simulink library "newton"  (R2023a)
settings: Solver=VariableStepAuto  StartTime=0.0  StopTime=10.0  RelTol=1e-3
undefined symbols (not defined in the file): b, d, D_rot, D_transl, eulerlimit, g, J1, J2, J3, Jr, L, m, R
settings Model: Creator=Alex  LastModifiedBy=Alex

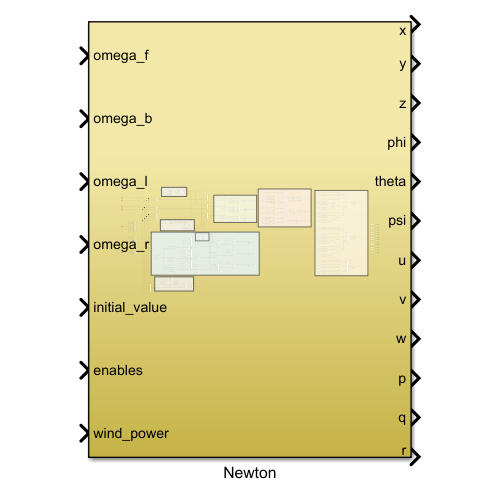
[thumbnail: Simulink's stored preview of the top-level diagram]
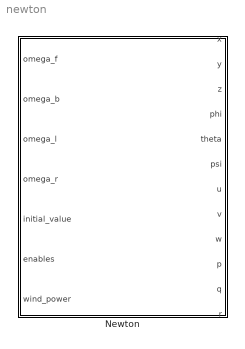
== system newton ==
  Newton : Subsystem

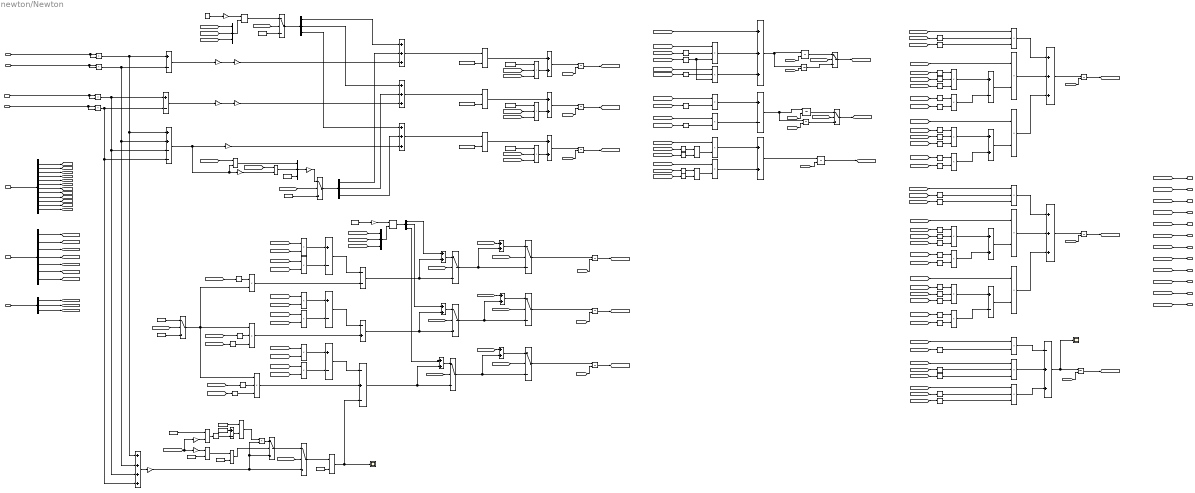
== system newton/Newton ==
  note: Drag force
  note: Ground
  note: Drag torque
  note: Gyro
  note: Inertial velocities in terms of body fixed velocities
      | Translational velocities
  note: Newton's second law
      | Translational accelerations
  note: Euler Angles
      | Rotational velocities
  note: Euler equations of motion
      | Rotational accelerations
  omega_f : Inport
  omega_b : Inport  Port=2
  omega_l : Inport  Port=3
  omega_r : Inport  Port=4
  initial_value : Inport  Port=5
  enables : Inport  Port=6
  wind_power : Inport  Port=7
  Add{,1,8,15..17,19,23,26} (9 alike) : Sum  Inputs=+-
  Add{7,10..11,18,21,25} (6 alike) : Sum  Inputs=+++
  Add12 : Sum  Inputs=--
  Add13 : Sum  Inputs=-+
  Add14 : Sum  Inputs=-+-
  Add2 : Sum  Inputs=++--
  Add{3..5,9,20,22,27..32} (12 alike) : Sum
  Add24 : Sum  Inputs=-++
  Add6 : Sum  Inputs=++++
  Constant : Constant  Value=J1
  Constant1 : Constant  Value=J2
  Constant10 : Constant  Value=R
  Constant{7,9,11,13} (4 alike) : Constant  Value=0
  Constant12 : Constant  Value=D_rot
  Constant14 : Constant  Value=0.25
  Constant15 : Constant  Value=R
  Constant16 : Constant
  Constant17 : Constant
  Constant18 : Constant  Value=D_transl
  Constant2 : Constant  Value=J3
  Constant3 : Constant  Value=(J2-J3)/J1
  Constant4 : Constant  Value=(J3-J1)/J2
  Constant5 : Constant  Value=(J1-J2)/J3
  Constant6 : Constant  Value=m
  Constant8 : Constant  Value=g
  Cos10 : Trigonometry
  Cos{2..8,11..12} (9 alike) : Trigonometry  Operator=cos
  Cos13 : Trigonometry
  Cos9 : Trigonometry
  Demux : Demux  Outputs=12
  Demux1 : Demux  Outputs=7
  Demux{2..5} (4 alike) : Demux  Outputs=3
  Divide{,1..8} (9 alike) : Product  Inputs=*/
  Gain : Gain  Gain=b
  Gain1 : Gain  Gain=L
  Gain10 : Gain  Gain=4
  Gain{6,8..9,11} (4 alike) : Gain  Gain=-1
  Gain2 : Gain  Gain=b
  Gain3 : Gain  Gain=L
  Gain4 : Gain  Gain=d
  Gain5 : Gain  Gain=b
  Gain7 : Gain  Gain=Jr
  Integrator{,1..3,6..7,9..13} (11 alike) : Integrator  InitialConditionSource=external
  Integrator4 : Integrator  InitialConditionSource=external  LimitOutput=on  UpperSaturationLimit=eulerlimit  LowerSaturationLimit=-eulerlimit
  Integrator5 : Integrator  InitialConditionSource=external  LimitOutput=on  UpperSaturationLimit=eulerlimit  LowerSaturationLimit=-eulerlimit
  Integrator8 : Integrator  InitialConditionSource=external  LimitOutput=on  UpperSaturationLimit=pi  LowerSaturationLimit=-pi
  Mux : Mux  Inputs=3
  Mux1 : Mux  Inputs=3
  Mux2 : Mux  Inputs=3
  Product{,1..3,9..13,17..19,21..26,28..29,31,33,35..36,38,40,42} (27 alike) : Product
  Product{4..8,14..15,27,30,32,34,37,39,41,43} (15 alike) : Product  Inputs=3
  Product16 : Product  Multiplication=Matrix(*)
  Product20 : Product  Multiplication=Matrix(*)
  Relational Operator : RelationalOperator  Operator=>  OutDataTypeStr=boolean  RndMeth=Simplest  InputSameDT=off
  Scope1 : Scope
  Scope6 : Scope
  Sin{,3..4,8,10,12..19,21..22,24..25} (17 alike) : Trigonometry
  Sin{1..2,5..7,9,11,20,23,26..29} (13 alike) : Trigonometry  Operator=cos
  Square : Math  Operator=square
  Switch{,1..12} (13 alike) : Switch  Criteria=u2 ~= 0  SaturateOnIntegerOverflow=off  InputSameDT=off
  Tan : Trigonometry  Operator=tan
  x : Outport
  y : Outport  Port=2
  z : Outport  Port=3
  phi : Outport  Port=4
  theta : Outport  Port=5
  psi : Outport  Port=6
  u : Outport  Port=7
  v : Outport  Port=8
  w : Outport  Port=9
  p : Outport  Port=10
  q : Outport  Port=11
  r : Outport  Port=12
  wires:
  omega_l/1 -> Product/2, Product/1
  omega_r/1 -> Product1/2, Product1/1
  Product/1 -> Add6/1, Add2/1, Add/1
  Product1/1 -> Add6/2, Add2/2, Add/2
  Add/1 -> Gain/1
  Gain/1 -> Gain1/1
  Gain1/1 -> Add25/3  "M1"
  Gain3/1 -> Add11/3  "M2"
  Gain2/1 -> Gain3/1
  Add1/1 -> Gain2/1
  Product3/1 -> Add1/2, Add6/4, Add2/4
  Product2/1 -> Add1/1, Add6/3, Add2/3
  omega_b/1 -> Product3/2, Product3/1
  omega_f/1 -> Product2/2, Product2/1
  Add2/1 -> Gain8/1, Product17/2, Gain4/1
  Gain4/1 -> Add10/3  "M3"
  Constant/1 -> Divide/2
  Constant1/1 -> Divide1/2
  Constant2/1 -> Divide2/2
  Divide/1 -> Add3/1
  Divide1/1 -> Add4/1
  Divide2/1 -> Add5/1
  Integrator/1 -> [p]  "p"
  Integrator1/1 -> [q]  "q"
  Integrator2/1 -> [r]  "r"
  Product4/1 -> Add3/2
  Product5/1 -> Add4/2
  Product6/1 -> Add5/2
  Constant3/1 -> Product4/1
  Constant4/1 -> Product5/1
  Constant5/1 -> Product6/1
  Add3/1 -> Integrator/1
  Add4/1 -> Integrator1/1
  Add5/1 -> Integrator2/1
  [q] -> Product4/2
  [r] -> Product4/3
  [r] -> Product5/2
  [p] -> Product5/3
  [p] -> Product6/2
  [q] -> Product6/3
  Add6/1 -> Gain5/1
  Gain5/1 -> Product19/2, Switch4/3, Switch2/3  "Fa"
  [p] -> Add7/1
  Product7/1 -> Add7/2
  Product8/1 -> Add7/3
  [phi] -> Sin/1
  Sin/1 -> Product7/2
  [theta] -> Tan/1
  Tan/1 -> Product8/3, Product7/3
  [phi] -> Sin1/1
  Sin1/1 -> Product8/2
  [r] -> Product8/1
  [phi] -> Sin2/1
  Sin2/1 -> Product9/2
  [q] -> Product9/1
  Product9/1 -> Add8/1
  Product10/1 -> Add8/2
  [r] -> Product10/1
  [phi] -> Sin3/1
  Sin3/1 -> Product10/2
  Divide3/1 -> Product11/2
  [q] -> Product11/1
  [r] -> Product12/1
  [phi] -> Sin4/1
  Sin4/1 -> Divide3/1
  Sin5/1 -> Divide3/2
  [theta] -> Sin5/1
  Product11/1 -> Add9/1
  Product12/1 -> Add9/2
  Divide4/1 -> Product12/2
  [phi] -> Sin6/1
  Sin6/1 -> Divide4/1
  Sin7/1 -> Divide4/2
  [theta] -> Sin7/1
  Constant6/1 -> Divide5/2
  Product14/1 -> Add13/2
  Product13/1 -> Add12/2
  Product21/1 -> Add15/1
  Product22/1 -> Add15/2
  Add15/1 -> Add12/1
  Switch10/1 -> Integrator12/1
  Integrator12/1 -> [u]  "u"
  Switch9/1 -> Integrator6/1
  Integrator6/1 -> [v]  "v"
  Integrator7/1 -> [w]  "w"
  [w] -> Product21/2
  [q] -> Product21/1
  [r] -> Product22/1
  [v] -> Product22/2
  Add16/1 -> Add13/1
  [w] -> Product24/2
  [p] -> Product24/1
  [r] -> Product23/1
  [u] -> Product23/2
  Product24/1 -> Add16/2
  Product23/1 -> Add16/1
  Product25/1 -> Add17/1
  Product26/1 -> Add17/2
  [v] -> Product25/2
  [p] -> Product25/1
  [q] -> Product26/1
  [u] -> Product26/2
  Add17/1 -> Add14/1
  Product28/1 -> Add18/2
  Product27/1 -> Add18/1
  Product29/1 -> Add18/3
  [u] -> Product27/1
  [v] -> Product28/1
  [w] -> Product29/1
  Integrator10/1 -> [x]
  Add19/1 -> Product28/2
  Add20/1 -> Product29/2
  [theta] -> Cos2/1
  Cos2/1 -> Product27/2
  [psi] -> Cos3/1
  Cos3/1 -> Product27/3
  Product30/1 -> Add19/1
  Sin12/1 -> Product30/1
  [phi] -> Sin12/1
  Sin13/1 -> Product30/2
  [theta] -> Sin13/1
  [psi] -> Cos4/1
  Cos4/1 -> Product30/3
  Product31/1 -> Add19/2
  Sin14/1 -> Product31/2
  [phi] -> Cos5/1
  [psi] -> Sin14/1
  Cos5/1 -> Product31/1
  Product32/1 -> Add20/1
  Product33/1 -> Add20/2
  Cos6/1 -> Product32/1
  Sin15/1 -> Product32/2
  Cos7/1 -> Product32/3
  [phi] -> Cos6/1
  [theta] -> Sin15/1
  [psi] -> Cos7/1
  Sin16/1 -> Product33/1
  Sin17/1 -> Product33/2
  [phi] -> Sin16/1
  [psi] -> Sin17/1
  [psi] -> Sin23/1
  [phi] -> Sin22/1
  Sin23/1 -> Product40/2
  Sin22/1 -> Product40/1
  [psi] -> Cos13/1
  [theta] -> Sin21/1
  [phi] -> Cos12/1
  Cos13/1 -> Product39/3
  Sin21/1 -> Product39/2
  Cos12/1 -> Product39/1
  Product40/1 -> Add23/2
  Product39/1 -> Add23/1
  Cos11/1 -> Product38/1
  [psi] -> Sin20/1
  [phi] -> Cos11/1
  Sin20/1 -> Product38/2
  Product38/1 -> Add22/2
  Cos10/1 -> Product37/3
  [psi] -> Cos10/1
  [theta] -> Sin19/1
  Sin19/1 -> Product37/2
  [phi] -> Sin18/1
  Sin18/1 -> Product37/1
  Product37/1 -> Add22/1
  Cos9/1 -> Product34/3
  [psi] -> Cos9/1
  Cos8/1 -> Product34/2
  [theta] -> Cos8/1
  Add23/1 -> Product36/2
  Add22/1 -> Product35/2
  Integrator11/1 -> [y]
  [w] -> Product36/1
  [v] -> Product35/1
  [u] -> Product34/1
  Product36/1 -> Add21/3
  Product34/1 -> Add21/1
  Product35/1 -> Add21/2
  Add24/1 -> Integrator3/1, Scope6/1
  Integrator3/1 -> [z]
  Product41/1 -> Add24/3
  Product43/1 -> Add24/2
  Product42/1 -> Add24/1
  [theta] -> Sin24/1
  [u] -> Product42/1
  Sin24/1 -> Product42/2
  [v] -> Product43/1
  [w] -> Product41/1
  [phi] -> Sin27/1
  [theta] -> Sin28/1
  [phi] -> Sin25/1
  [theta] -> Sin26/1
  Sin25/1 -> Product43/2
  Sin26/1 -> Product43/3
  Sin27/1 -> Product41/2
  Sin28/1 -> Product41/3
  [x] -> x/1
  [y] -> y/1
  [r] -> r/1
  [q] -> q/1
  [p] -> p/1
  [w] -> w/1
  [v] -> v/1
  [u] -> u/1
  [psi] -> psi/1
  [theta] -> theta/1
  [phi] -> phi/1
  [z] -> z/1
  Divide5/1 -> Scope1/1, Add14/3
  [q] -> Product7/1
  [theta] -> Sin8/1
  Sin8/1 -> Product13/1
  Switch/1 -> Product14/1, Product13/2, Product15/1  "gravity"
  [theta] -> Sin9/1
  Sin9/1 -> Product14/2
  [phi] -> Sin10/1
  Sin10/1 -> Product14/3
  Product15/1 -> Add14/2
  [theta] -> Sin11/1
  Sin11/1 -> Product15/2
  Sin29/1 -> Product15/3
  [phi] -> Sin29/1
  initial_value/1 -> Demux/1
  Demux/1 -> [x0]
  Demux/2 -> [y0]
  Demux/3 -> [z0]
  Demux/4 -> [phi0]
  Demux/5 -> [theta0]
  Demux/6 -> [psi0]
  Demux/7 -> [u0]
  Demux/8 -> [v0]
  Demux/9 -> [w0]
  Demux/10 -> [p0]
  Demux/11 -> [q0]
  Demux/12 -> [r0]
  [p0] -> Integrator/2
  [q0] -> Integrator1/2
  [r0] -> Integrator2/2
  [u0] -> Integrator12/2
  [v0] -> Integrator6/2
  [w0] -> Integrator7/2
  Switch8/1 -> Integrator7/1
  [z0] -> Integrator3/2
  [y0] -> Integrator11/2
  Add21/1 -> Integrator11/1
  Add18/1 -> Integrator10/1
  [x0] -> Integrator10/2
  enables/1 -> Demux1/1
  Demux1/1 -> [Ena_gravity]
  Demux1/3 -> [Ena_gyro]
  Demux1/4 -> [Ena_ground]
  Demux1/5 -> [Ena_drag_force]
  Demux1/6 -> [Ena_drag_torque]
  Demux1/7 -> [Ena_wind]
  wind_power/1 -> Demux5/1
  [Ena_gravity] -> Switch/2
  Constant8/1 -> Switch/1
  Constant7/1 -> Switch/3
  Add10/1 -> Divide2/1  "tau3"
  Add11/1 -> Divide1/1  "tau2"
  Add25/1 -> Divide/1  "tau1"
  [Ena_gyro] -> Switch1/2
  [Ena_drag_torque] -> Switch3/2
  Constant9/1 -> Switch3/3
  Constant11/1 -> Switch1/3
  Constant12/1 -> Gain6/1
  Gain6/1 -> Product16/1
  [q] -> Mux/2
  [p] -> Mux/1
  [r] -> Mux/3
  Mux/1 -> Product16/2
  Product16/1 -> Switch3/1
  Switch3/1 -> Demux2/1  "drag_torque"
  Switch1/1 -> Demux3/1  "gyro"
  [q] -> Product17/1
  [p] -> Product18/1
  Product17/1 -> Mux1/1
  Product18/1 -> Mux1/2
  Constant13/1 -> Mux1/3
  Mux1/1 -> Gain7/1
  Gain7/1 -> Switch1/1
  Gain8/1 -> Product18/2
  Demux3/3 -> Add10/2
  Demux3/2 -> Add11/2
  Demux3/1 -> Add25/2
  Demux2/2 -> Add11/1
  [Ena_ground] -> Switch2/2
  Switch2/1 -> Divide5/1  "ground"
  Switch4/1 -> Switch2/1
  [z] -> Gain10/1, Gain9/1
  Gain9/1 -> Divide6/1
  Divide6/1 -> Relational Operator/1
  Constant10/1 -> Divide6/2
  Relational Operator/1 -> Switch4/2
  Constant14/1 -> Relational Operator/2
  Product19/1 -> Switch4/1
  Constant15/1 -> Divide7/1
  Gain10/1 -> Divide7/2
  Divide7/1 -> Square/1
  Square/1 -> Add26/2
  Constant16/1 -> Add26/1
  Divide8/1 -> Product19/1
  Add26/1 -> Divide8/2
  Constant17/1 -> Divide8/1
  [Ena_drag_force] -> Switch5/2
  Add14/1 -> Add27/2, Switch5/3
  Add27/1 -> Switch5/1
  Mux2/1 -> Product20/2
  [w] -> Mux2/3
  [u] -> Mux2/1
  Gain11/1 -> Product20/1
  Constant18/1 -> Gain11/1
  [v] -> Mux2/2
  Add28/1 -> Switch6/1
  Add13/1 -> Switch6/3, Add28/2
  [Ena_drag_force] -> Switch6/2
  [Ena_drag_force] -> Switch7/2
  Add12/1 -> Add29/2, Switch7/3
  Add29/1 -> Switch7/1
  Product20/1 -> Demux4/1
  Demux4/2 -> Add28/1
  Demux4/3 -> Add27/1
  Demux2/1 -> Add25/1
  Demux2/3 -> Add10/1
  Switch5/1 -> Add32/2, Switch8/3
  Switch6/1 -> Add31/2, Switch9/3
  Switch7/1 -> Add30/2, Switch10/3
  [Ena_wind] -> Switch9/2
  [Ena_wind] -> Switch8/2
  [Ena_wind] -> Switch10/2
  Add30/1 -> Switch10/1
  Add31/1 -> Switch9/1
  Add32/1 -> Switch8/1
  Demux5/1 -> [wind_x]
  Demux5/2 -> [wind_y]
  Demux5/3 -> [wind_z]
  [wind_x] -> Add30/1
  [wind_y] -> Add31/1
  [wind_z] -> Add32/1
  Demux4/1 -> Add29/1
  Demux1/2 -> [Ena_euler_sat]
  Add7/1 -> Integrator13/1, Integrator4/1  "phidot"
  Add8/1 -> Integrator9/1, Integrator5/1  "thetadot"
  [phi0] -> Integrator13/2
  [theta0] -> Integrator5/2
  Integrator4/1 -> Switch12/1  "phi_lim"
  [Ena_euler_sat] -> Switch12/2
  Add9/1 -> Integrator8/1  "psidot"
  Switch12/1 -> [phi]  "phi"
  Integrator9/1 -> Switch11/3  "theta_nolim"
  Integrator8/1 -> [psi]  "psi"
  [theta0] -> Integrator9/2
  Switch11/1 -> [theta]  "theta"
  [Ena_euler_sat] -> Switch11/2
  Integrator5/1 -> Switch11/1  "theta_lim"
  Integrator13/1 -> Switch12/3  "phi_nolim"
  [phi0] -> Integrator4/2
  [psi0] -> Integrator8/2
